simulink model "ex19_5"  (R2023a)
settings: Solver=VariableStepAuto  StartTime=0.0  StopTime=3.6e-3  FixedStep=1/(2.5e3)  RelTol=1e-6
undefined symbols (not defined in the file or in its folder): K, p
libraries: spsTriangleGeneratorLib x1
settings Model: Creator=eechris  LastModifiedBy=eechris

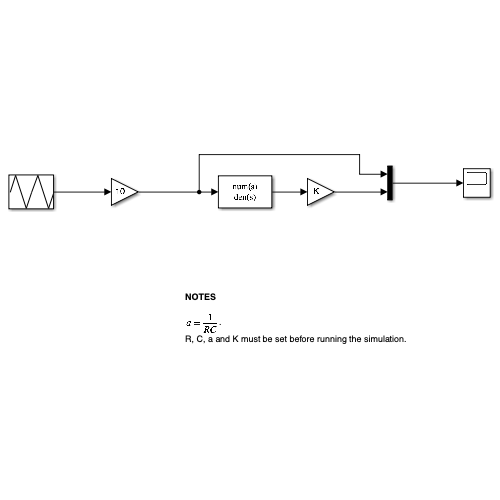
[thumbnail: Simulink's stored preview of the top-level diagram]
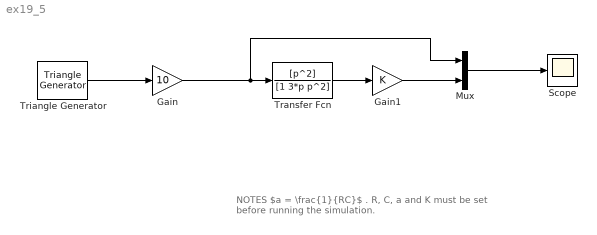
== system ex19_5 ==
  note: NOTES
      |
      | $a = \frac{1}{RC}$ .
      | R, C, a and K must be set before running the simulation.
  Gain : Gain  Gain=10
  Gain1 : Gain  Gain=K
  Mux : Mux  Inputs=2
  Scope : Scope
  Transfer Fcn : TransferFcn  Numerator=[p^2]  Denominator=[1 3*p p^2]
  Triangle Generator : spsTriangleGeneratorLib/Triangle Generator  Freq=2.5e3  Phase=90  Ts=0
  wires:
  Triangle Generator/1 -> Gain/1
  Gain/1 -> Transfer Fcn/1, Mux/1
  Transfer Fcn/1 -> Gain1/1
  Mux/1 -> Scope/1
  Gain1/1 -> Mux/2
